simulink model "OMAP"  (R2018b)
settings: Solver=FixedStepDiscrete  StartTime=0.0  StopTime=10.0  FixedStep=0.01  RelTol=1e-3
values from neighbouring files (symbols this model uses):
  Clb_ICADirect_LaneDisp_StateFive = Simulink.Parameter    [omap_ver_442.m]
  Clb_ICADirect_LaneDisp_StateFour = Simulink.Parameter    [omap_ver_442.m]
  Clb_ICADirect_LaneDisp_StateOne = Simulink.Parameter    [omap_ver_442.m]
  Clb_ICADirect_LaneDisp_StateThree = Simulink.Parameter    [omap_ver_442.m]
  Clb_ICADirect_LaneDisp_StateTwo = Simulink.Parameter    [omap_ver_442.m]
  Clb_ICADirect_LaneDisp_StateZero = Simulink.Parameter    [omap_ver_442.m]
  Clb_ICADirect_LaneDispSW = Simulink.Parameter    [omap_ver_442.m]
  Clb_ICADirect_TrnLghtsCom_Switch = Simulink.Parameter    [omap_ver_442.m]
  Clb_ICADirect_TrnLghtsCom_Value = Simulink.Parameter    [omap_ver_442.m]
  Clb_ICADirect_TrnLghtsCrtl_Inhb = Simulink.Parameter    [omap_ver_442.m]
  OMAP_ACCAEB_EMSESC_Decel = Simulink.Parameter    [omap_ver_442.m]
  OMAP_ACCFCW_IC_Decel = Simulink.Parameter    [omap_ver_442.m]
  OMAP_clb_ACC_RVVReqType = Simulink.Parameter    [omap_ver_442.m]
  OMAP_clb_ACC_RVVReqType_Switch = Simulink.Parameter    [omap_ver_442.m]
  OMAP_clb_ACCHeadwayDisplay = Simulink.Parameter    [omap_ver_442.m]
  OMAP_clb_ACCHeadwayDisplay_Switch = Simulink.Parameter    [omap_ver_442.m]
  OMAP_clb_ACCHeadwayIcon = Simulink.Parameter    [omap_ver_442.m]
  OMAP_clb_ACCHeadwayIcon_Switch = Simulink.Parameter    [omap_ver_442.m]
  OMAP_clb_ACCMessagePrompt = Simulink.Parameter    [omap_ver_442.m]
  OMAP_clb_ACCMessagePrompt_Switch = Simulink.Parameter    [omap_ver_442.m]
  OMAP_clb_ACCRequestEPB = Simulink.Parameter    [omap_ver_442.m]
  OMAP_clb_ACCRequestEPB_Switch = Simulink.Parameter    [omap_ver_442.m]
  OMAP_clb_ACCSetSpeed = Simulink.Parameter    [omap_ver_442.m]
  OMAP_clb_ACCSetSpeed_Switch = Simulink.Parameter    [omap_ver_442.m]
  OMAP_clb_ACCSetSpeedDis = Simulink.Parameter    [omap_ver_442.m]
  OMAP_clb_ACCSetSpeedDis_Switch = Simulink.Parameter    [omap_ver_442.m]
  OMAP_clb_ACCState = Simulink.Parameter    [omap_ver_442.m]
  OMAP_clb_ACCState_Switch = Simulink.Parameter    [omap_ver_442.m]
  OMAP_clb_ACCStatusIconDis = Simulink.Parameter    [omap_ver_442.m]
  OMAP_clb_ACCStatusIconDis_Switch = Simulink.Parameter    [omap_ver_442.m]
  OMAP_clb_ACCTorqueReq = Simulink.Parameter    [omap_ver_442.m]
  OMAP_clb_ACCTorqueReq_Switch = Simulink.Parameter    [omap_ver_442.m]
  OMAP_clb_ADAS_State = Simulink.Parameter    [omap_ver_442.m]
  OMAP_clb_ADAS_State_Switch = Simulink.Parameter    [omap_ver_442.m]
  OMAP_clb_AEBAlertReq = Simulink.Parameter    [omap_ver_442.m]
  OMAP_clb_AEBAlertReq_Switch = Simulink.Parameter    [omap_ver_442.m]
  OMAP_clb_AEBBrakingProg = Simulink.Parameter    [omap_ver_442.m]
  OMAP_clb_AEBBrakingProg_Switch = Simulink.Parameter    [omap_ver_442.m]
  OMAP_clb_AEBFaultStatus = Simulink.Parameter    [omap_ver_442.m]
  OMAP_clb_AEBFaultStatus_Switch = Simulink.Parameter    [omap_ver_442.m]
  OMAP_clb_AEBMassageDisp = Simulink.Parameter    [omap_ver_442.m]
  OMAP_clb_AEBMassageDisp_Switch = Simulink.Parameter    [omap_ver_442.m]
  OMAP_clb_AEBState = Simulink.Parameter    [omap_ver_442.m]
  OMAP_clb_AEBState_Switch = Simulink.Parameter    [omap_ver_442.m]
  OMAP_clb_AEBSwitchStatus = Simulink.Parameter    [omap_ver_442.m]
  OMAP_clb_AEBSwitchStatus_Switch = Simulink.Parameter    [omap_ver_442.m]
  OMAP_clb_BrakeRequest = Simulink.Parameter    [omap_ver_442.m]
  OMAP_clb_BrakeRequest_Switch = Simulink.Parameter    [omap_ver_442.m]
  OMAP_clb_DecelerationSet = Simulink.Parameter    [omap_ver_442.m]
  OMAP_clb_DecelerationSet_Switch = Simulink.Parameter    [omap_ver_442.m]
  OMAP_clb_DecelerationType = Simulink.Parameter    [omap_ver_442.m]
  OMAP_clb_DecelerationType_Switch = Simulink.Parameter    [omap_ver_442.m]
  OMAP_clb_DeclControlReq = Simulink.Parameter    [omap_ver_442.m]
  OMAP_clb_DeclControlReq_Switch = Simulink.Parameter    [omap_ver_442.m]
  OMAP_clb_DownorUpGearMinTime = Simulink.Parameter    [omap_ver_442.m]
  OMAP_clb_DownorUpGearMinTime_Switch = Simulink.Parameter    [omap_ver_442.m]
  OMAP_clb_ELKPopupMessage = Simulink.Parameter    [omap_ver_442.m]
  OMAP_clb_ELKPopupMessage_Switch = Simulink.Parameter    [omap_ver_442.m]
  OMAP_clb_ELKSts = Simulink.Parameter    [omap_ver_442.m]
  OMAP_clb_ELKSts_Switch = Simulink.Parameter    [omap_ver_442.m]
  OMAP_clb_ESAFaultSt = Simulink.Parameter    [omap_ver_442.m]
  OMAP_clb_ESAFaultSt_Switch = Simulink.Parameter    [omap_ver_442.m]
  OMAP_clb_ESARequest = Simulink.Parameter    [omap_ver_442.m]
  OMAP_clb_ESARequest_Switch = Simulink.Parameter    [omap_ver_442.m]
  OMAP_clb_ESAState = Simulink.Parameter    [omap_ver_442.m]
  OMAP_clb_ESAState_Switch = Simulink.Parameter    [omap_ver_442.m]
  OMAP_clb_ESATorqueReq = Simulink.Parameter    [omap_ver_442.m]
  OMAP_clb_ESATorqueReq_Switch = Simulink.Parameter    [omap_ver_442.m]
  OMAP_clb_ESCDriveOff = Simulink.Parameter    [omap_ver_442.m]
  OMAP_clb_ESCDriveOff_Switch = Simulink.Parameter    [omap_ver_442.m]
  OMAP_clb_ESCHoldReq = Simulink.Parameter    [omap_ver_442.m]
  OMAP_clb_ESCHoldReq_Switch = Simulink.Parameter    [omap_ver_442.m]
  OMAP_clb_Handsoffwarning = Simulink.Parameter    [omap_ver_442.m]
  OMAP_clb_Handsoffwarning_Switch = Simulink.Parameter    [omap_ver_442.m]
  OMAP_clb_HapticAlarmReq = Simulink.Parameter    [omap_ver_442.m]
  OMAP_clb_HapticAlarmReq_Switch = Simulink.Parameter    [omap_ver_442.m]
  OMAP_clb_HMIPopupMassage = Simulink.Parameter    [omap_ver_442.m]
  OMAP_clb_HMIPopupMassage_Switch = Simulink.Parameter    [omap_ver_442.m]
  OMAP_clb_HWAActionSts = Simulink.Parameter    [omap_ver_442.m]
  OMAP_clb_HWAActionSts_Switch = Simulink.Parameter    [omap_ver_442.m]
  OMAP_clb_HWAMode = Simulink.Parameter    [omap_ver_442.m]
  OMAP_clb_HWAMode_Switch = Simulink.Parameter    [omap_ver_442.m]
  OMAP_clb_HWATurnOnIdctr = Simulink.Parameter    [omap_ver_442.m]
  OMAP_clb_HWATurnOnIdctr_Switch = Simulink.Parameter    [omap_ver_442.m]
  OMAP_clb_ICAMassageDisp = Simulink.Parameter    [omap_ver_442.m]
  OMAP_clb_ICAMassageDisp_Switch = Simulink.Parameter    [omap_ver_442.m]
  OMAP_clb_ICAStatusIcon = Simulink.Parameter    [omap_ver_442.m]
  OMAP_clb_ICAStatusIcon_Switch = Simulink.Parameter    [omap_ver_442.m]
  OMAP_clb_ISLCDriverRemind = Simulink.Parameter    [omap_ver_442.m]
  OMAP_clb_ISLCDriverRemind_Switch = Simulink.Parameter    [omap_ver_442.m]
  OMAP_clb_ISLCState = Simulink.Parameter    [omap_ver_442.m]
  OMAP_clb_ISLCState_Switch = Simulink.Parameter    [omap_ver_442.m]
  OMAP_clb_JAFaultSt = Simulink.Parameter    [omap_ver_442.m]
  OMAP_clb_JAFaultSt_Switch = Simulink.Parameter    [omap_ver_442.m]
  OMAP_clb_LCAPopupMessage = Simulink.Parameter    [omap_ver_442.m]
  OMAP_clb_LCAPopupMessage_Switch = Simulink.Parameter    [omap_ver_442.m]
  OMAP_clb_LCAStatusDisplay = Simulink.Parameter    [omap_ver_442.m]
  OMAP_clb_LCAStatusDisplay_Switch = Simulink.Parameter    [omap_ver_442.m]
  OMAP_clb_LDWStatusDisplay = Simulink.Parameter    [omap_ver_442.m]
  OMAP_clb_LDWStatusDisplay_Switch = Simulink.Parameter    [omap_ver_442.m]
  OMAP_clb_LDWWarningSt = Simulink.Parameter    [omap_ver_442.m]
  OMAP_clb_LDWWarningSt_Switch = Simulink.Parameter    [omap_ver_442.m]
  OMAP_clb_LightControlValid = Simulink.Parameter    [omap_ver_442.m]
  OMAP_clb_LightControlValid_Switch = Simulink.Parameter    [omap_ver_442.m]
  OMAP_clb_LKAActivation = Simulink.Parameter    [omap_ver_442.m]
  OMAP_clb_LKAActivation_Switch = Simulink.Parameter    [omap_ver_442.m]
  OMAP_clb_LKAAngleReq = Simulink.Parameter    [omap_ver_442.m]
  OMAP_clb_LKAAngleReq_Switch = Simulink.Parameter    [omap_ver_442.m]
  OMAP_clb_LKAMode = Simulink.Parameter    [omap_ver_442.m]
  OMAP_clb_LKAMode_Switch = Simulink.Parameter    [omap_ver_442.m]
  OMAP_clb_LKAorELK_CoolTime = Simulink.Parameter    [omap_ver_442.m]
  OMAP_clb_LKAState = Simulink.Parameter    [omap_ver_442.m]
  OMAP_clb_LKAState_Switch = Simulink.Parameter    [omap_ver_442.m]
  OMAP_clb_LKAStatusDisplay = Simulink.Parameter    [omap_ver_442.m]
  OMAP_clb_LKAStatusDisplay_Switch = Simulink.Parameter    [omap_ver_442.m]
  OMAP_clb_LKASwitchState = Simulink.Parameter    [omap_ver_442.m]
  OMAP_clb_LKASwitchState_Switch = Simulink.Parameter    [omap_ver_442.m]
  OMAP_clb_LKATorqFactReq = Simulink.Parameter    [omap_ver_442.m]
  OMAP_clb_LKATorqFactReq_Switch = Simulink.Parameter    [omap_ver_442.m]
  OMAP_clb_PrefillRequest = Simulink.Parameter    [omap_ver_442.m]
  ... (+36 more)
libraries: simulink x184, canmsglib x2
(part 8 of 14)

== system OMAP/Runnable_OMAP_10ms_sys/OMAP_Module/ACCS_Direct/ACCS_Define/Human_Machine_Interface(ACC_HMI) ==
  CIPV_ID_Longitudinal_Distance : Inport
  CIPV_ID : Inport  Port=2
  ACC_State : Inport  Port=3
  ACCActive_Signal : Inport  Port=4
  ACC_ICA_Flag : Inport  Port=5
  HeadWaySet : Inport  Port=6
  VelocitySet : Inport  Port=7
  ACC_go_request : Inport  Port=8
  ACC_DecReq : Inport  Port=9
  Bus Selector : BusSelector  OutputSignals=ACC_Vehicle_Icon_Display,ACC_Set_Speed_Display,ACC_DesiredHeadway_Icon_Basic,RVVACC_Vehiclespeed_request_type
  Gain : Gain  OutDataTypeStr=uint8
  Gain1 : Gain  OutDataTypeStr=uint8
  Subsystem : Subsystem
  Subsystem9 : Subsystem
  Text_PopUp : Subsystem
  ACC_DesiredHeadway_Display : Outport
  ACC_DesiredHeadway_Icon_Basic : Outport  Port=2
  ACC_Desired_Set_Speed : Outport  Port=3
  ACC_Set_Speed_Display : Outport  Port=4
  ACC_Vehicle_Icon_Display : Outport  Port=5
  RVVACC_Vehiclespeed_request_type : Outport  Port=6
  ACC_Pop_Up_Message : Outport  Port=7
  ACC_HMI_TgDisp_Flag : Outport  Port=8
  TARGET_POSITION : Outport  Port=9
  ACC_Pop_Up_Message_TJA : Outport  Port=10
  wires:
  VelocitySet/1 -> Gain/1, Subsystem9/3(VelocitySet)
  HeadWaySet/1 -> Gain1/1
  Subsystem9/1(Out1) -> Bus Selector/1
  Gain/1 -> ACC_Desired_Set_Speed/1  "ACC_Desired_Set_Speed"
  CIPV_ID_Longitudinal_Distance/1 -> Subsystem/1(Distance)
  Subsystem/2(TgDisp_Flag) -> ACC_HMI_TgDisp_Flag/1  "ACC_HMI_TgDisp_Flag"
  Subsystem/1(TARGET_POSITION) -> TARGET_POSITION/1  "TARGET_POSITION"
  CIPV_ID/1 -> Subsystem/2(CIPV_ID)
  Gain1/1 -> ACC_DesiredHeadway_Display/1  "ACC_DesiredHeadway_Display"
  Text_PopUp/1(For4F7) -> ACC_Pop_Up_Message/1  "ACC_Pop_Up_Message"
  Bus Selector/1 -> ACC_Vehicle_Icon_Display/1  "<ACC_Vehicle_Icon_Display>"
  Bus Selector/3 -> ACC_DesiredHeadway_Icon_Basic/1  "<ACC_DesiredHeadway_Icon_Basic>"
  Bus Selector/4 -> RVVACC_Vehiclespeed_request_type/1  "<RVVACC_Vehiclespeed_request_type>"
  Bus Selector/2 -> ACC_Set_Speed_Display/1  "<ACC_Set_Speed_Display>"
  ACCActive_Signal/1 -> Text_PopUp/3(ACCActive_Signal)
  Text_PopUp/2(ForTJA) -> ACC_Pop_Up_Message_TJA/1  "ACC_Pop_Up_Message_TJA"
  ACC_go_request/1 -> Text_PopUp/4(go_request)
  ACC_State/1 -> Subsystem9/1(ACC_State), Text_PopUp/1(ACC_State), Subsystem/3(ACC_State)
  ACC_ICA_Flag/1 -> Subsystem9/2(ACCICA_Flag), Text_PopUp/2(ACCICA_Flag)
  ACC_DecReq/1 -> Text_PopUp/5(ACC_DecReq)

== system OMAP/Runnable_OMAP_10ms_sys/OMAP_Module/ICA_Direct_G59/ICA_Define/ICA_EPS ==
  EPSPCEM_stICAState : Inport
  angle : Inport  Port=2
  torque_Req : Inport  Port=3
  torque : Inport  Port=4
  EPSPCEM_stEPSCtlState : Inport  Port=5
  Data Type Conversion : DataTypeConversion  OutDataTypeStr=uint16
  Data Type Conversion1 : DataTypeConversion  OutDataTypeStr=single
  Data Type Conversion2 : DataTypeConversion  OutDataTypeStr=uint16
  Data Type Conversion3 : DataTypeConversion  OutDataTypeStr=single
  Data Type Conversion4 : DataTypeConversion  OutDataTypeStr=single
  EPS_Ctr_Disable : Subsystem  TreatAsAtomicUnit=on
  EPS_Ctr_Enable : Subsystem  TreatAsAtomicUnit=on
  If1 : If  IfExpression=u1==3
  Merge{1..5} (5 alike) : Merge
  stEPS_State_Ctl_CMD : Outport
  LKA_TRQ_FACT_REQ : Outport  Port=2
  LKA_OR_LPA_REQ : Outport  Port=3
  ICA_STATE : Outport  Port=4
  ICABve_g_SteerAngleCmd_convert : Outport  Port=5
  ICABve_d_LKATorqueReq_convert : Outport  Port=6
  ICABve_g_LKATorqueReq_Value_convert : Outport  Port=7
  wires:
  Merge1/1 -> Data Type Conversion/1
  EPSPCEM_stEPSCtlState/1 -> EPS_Ctr_Disable/1(stEPSCtlState), EPS_Ctr_Enable/1(stEPSCtlState)
  EPS_Ctr_Enable/1(stEPSCtlCMD) -> Merge1/1
  If1/2 -> EPS_Ctr_Disable/Action
  EPS_Ctr_Enable/2(LKA_TRQ_FACT_REQ) -> Merge2/1
  EPS_Ctr_Disable/2(LKA_TRQ_FACT_REQ) -> Merge2/2
  Merge2/1 -> Data Type Conversion1/1
  EPSPCEM_stICAState/1 -> ICA_STATE/1, If1/1
  Data Type Conversion1/1 -> LKA_TRQ_FACT_REQ/1  "LKA_TRQ_FACT_REQ"
  EPS_Ctr_Disable/1(stEPSCtlCMD) -> Merge1/2
  If1/1 -> EPS_Ctr_Enable/Action
  Data Type Conversion/1 -> stEPS_State_Ctl_CMD/1
  EPS_Ctr_Enable/3(LKA_OR_LPA_REQ) -> Merge3/1
  Data Type Conversion2/1 -> LKA_OR_LPA_REQ/1
  Merge3/1 -> Data Type Conversion2/1
  EPS_Ctr_Disable/3(LKA_OR_LPA_REQ) -> Merge3/2
  Data Type Conversion3/1 -> ICABve_g_SteerAngleCmd_convert/1
  Merge5/1 -> Data Type Conversion4/1
  Merge4/1 -> Data Type Conversion3/1
  Data Type Conversion4/1 -> ICABve_g_LKATorqueReq_Value_convert/1
  EPS_Ctr_Disable/5(torque1) -> Merge5/2
  EPS_Ctr_Disable/4(angle1) -> Merge4/2
  angle/1 -> EPS_Ctr_Enable/2(angle)
  torque/1 -> EPS_Ctr_Enable/3(torque)
  EPS_Ctr_Enable/4(angle1) -> Merge4/1
  EPS_Ctr_Enable/5(torque1) -> Merge5/1
  torque_Req/1 -> ICABve_d_LKATorqueReq_convert/1

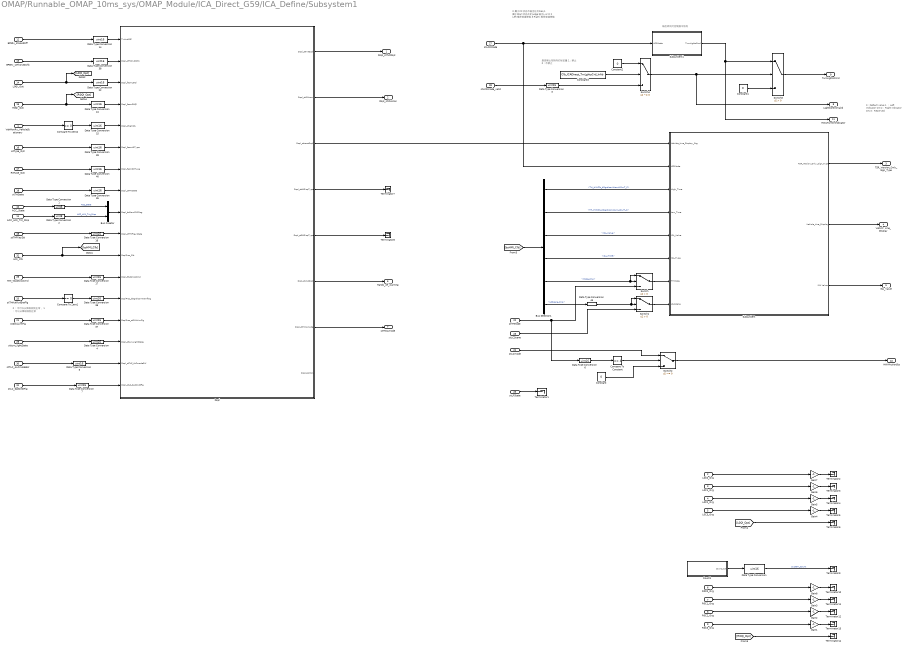
== system OMAP/Runnable_OMAP_10ms_sys/OMAP_Module/ICA_Direct_G59/ICA_Define/Subsystem1 ==
  note: 是否禁止控转向灯标定量
      | 1：禁止
      | 0：不禁止
  note: 0：Default value
      | 1：Left indicator ON
      | 2：Right indicator ON
      | 3：Reserved
  note: 输出转向灯控制指令信号
  note: 0 ：不可以从降级回到正常，
      | 1 ：可以从降级回到正常
  note: 0 属于CD状态不输出任何Req
      | 1 属于Start状态开始Judge输出L or R
      | 2 Left推荐变道使能
      | 3 Right 推荐变道使能
  VehMovRx_VehicleStationary : Inport
  L0C0_Org : Inport  Port=2
  L0C1_Org : Inport  Port=3
  L0C2_Org : Inport  Port=4
  L0C3_Org : Inport  Port=5
  R0C0_Org : Inport  Port=6
  R0C1_Org : Inport  Port=7
  R0C2_Org : Inport  Port=8
  R0C3_Org : Inport  Port=9
  ACC_State : Inport  Port=10
  ACC_HMI_Txt_Disp : Inport  Port=11
  EPSRx_stHandOff : Inport  Port=12
  EPSRx_stTkOvStChk : Inport  Port=13
  L0QI_Opt : Inport  Port=14
  R0QI_Opt : Inport  Port=15
  L0Type_Opt : Inport  Port=16
  R0Type_Opt : Inport  Port=17
  stTHState : Inport  Port=18
  stTHFKeyStt : Inport  Port=19
  stTHAutRydEnaFlg : Inport  Port=20
  stSWALimFlg : Inport  Port=21
  stTHMode : Inport  Port=22
  stLCScene : Inport  Port=23
  stLCmode : Inport  Port=24
  stLFState : Inport  Port=25
  HMI_tfAddVocCmd : Inport  Port=26
  stLCRMode : Inport  Port=27
  stLCRmode_valid : Inport  Port=28
  stturn_lightState : Inport  Port=29
  stTLC_ALCmodeSW : Inport  Port=30
  stLC_SpdCndtFlg : Inport  Port=31
  HMI_Clb : Inport  Port=32
  Bus Creator : BusCreator  Inputs=2
  Bus Selector1 : BusSelector  OutputSignals=TH_HMIClb_tiDgrdIconWarnHiDurT_C,TH_HMIClb_tiDgrdIconWarnLoDurT_C,ISA_Value,ISA_TYPE,Mode_tmp,LCScene_tmp
  Compare To Constant : simulink/Logic and Bit Operations/Compare To Constant  relop===  const=4  OutDataTypeStr=boolean
  Compare To Zero1 : simulink/Logic and Bit Operations/Compare To Zero  relop===  OutDataTypeStr=boolean
  Compare To Zero2 : simulink/Logic and Bit Operations/Compare To Zero  relop===  OutDataTypeStr=boolean
  Constant : Constant  Value=0  OutDataTypeStr=uint16
  Constant1 : Constant  Value=0  OutDataTypeStr=uint16
  Constant2 : Constant  Value=0  OutDataTypeStr=uint16
  Constant3 : Constant  Value=Clb_ICADirect_TrnLghtsCrtl_Inhb  OutDataTypeStr=uint16
  Count1 : MATLAB Function  TreatAsAtomicUnit=on
  Data Type Conversion{,3..7,14..17,22,24,35..40,45} (19 alike) : DataTypeConversion  OutDataTypeStr=uint16
  Data Type Conversion1 : DataTypeConversion  OutDataTypeStr=uint8
  Data Type Conversion2 : DataTypeConversion  OutDataTypeStr=uint8
  Dspl : Subsystem
  Gain{1..8} (8 alike) : Gain  Gain=-1  OutDataTypeStr=single
  Subsystem : Subsystem
  Subsystem1 : Subsystem
  Switch : Switch  Criteria=u2 > Threshold  OutDataTypeStr=uint16
  Switch1 : Switch  Criteria=u2 > Threshold  OutDataTypeStr=uint16
  Switch2 : Switch  Criteria=u2 ~= 0  OutDataTypeStr=uint16
  Switch3 : Switch  Criteria=u2 > Threshold  OutDataTypeStr=uint16
  Switch4 : Switch  Criteria=u2 ~= 0
  Terminator{1..14} (14 alike) : Terminator
  Dspl_stTxtDspl : Outport
  Dspl_stICAIcon : Outport  Port=2
  TSR_Version_Only_Sign_Type : Outport  Port=3
  Vehiclr_Line_Display : Outport  Port=4
  ISA_Value : Outport  Port=5
  Hands_off_warning : Outport  Port=6
  stHWAmode : Outport  Port=7
  LightControlValid : Outport  Port=8
  TurnLightsCmd : Outport  Port=9
  HWAActionSts : Outport  Port=10
  HWATurnOnIndicator : Outport  Port=11
  wires:
  R0C3_Org/1 -> Gain1/1
  L0C0_Org/1 -> Gain7/1
  stTHFKeyStt/1 -> Data Type Conversion16/1
  [L0QI_Opt] -> Terminator6/1
  Dspl/6(Dspl_stVocDspl) -> Hands_off_warning/1
  stLCScene/1 -> Switch1/3
  stTHMode/1 -> Data Type Conversion6/1, Switch/3
  L0QI_Opt/1 -> [L0QI_Opt], Data Type Conversion22/1
  stTHAutRydEnaFlg/1 -> Compare To Zero1/1
  stTHState/1 -> Data Type Conversion35/1
  stSWALimFlg/1 -> Data Type Conversion37/1
  [R0QI_Opt] -> Terminator14/1
  R0C0_Org/1 -> Gain8/1
  L0C2_Org/1 -> Gain5/1
  R0Type_Opt/1 -> Data Type Conversion40/1
  VehMovRx_VehicleStationary/1 -> Compare To Zero2/1
  Data Type Conversion24/1 -> Dspl/4(Dspl_facmR0Ql)
  R0QI_Opt/1 -> [R0QI_Opt], Data Type Conversion24/1
  R0C1_Org/1 -> Gain3/1
  Compare To Zero1/1 -> Data Type Conversion36/1
  Data Type Conversion39/1 -> Dspl/6(Dspl_facmL0Type)
  Data Type Conversion37/1 -> Dspl/14(DsplPrcs_stSWALimFlg)
  L0C3_Org/1 -> Gain4/1
  Data Type Conversion17/1 -> Dspl/12(Dspl_tfAddVocCmd)
  Bus Selector1/6 -> Data Type Conversion45/1  "<LCScene_tmp>"
  Data Type Conversion16/1 -> Dspl/10(Dspl_stTHFKeyState)
  EPSRx_stTkOvStChk/1 -> Data Type Conversion38/1
  [bsHMI_Clb] -> Bus Selector1/1
  Data Type Conversion45/1 -> Switch1/1, Switch1/2
  Data Type Conversion36/1 -> Dspl/13(DsplPrcs_dDgrdIconWarnflag)
  HMI_Clb/1 -> [bsHMI_Clb], Dspl/11(DsplPrcs_CIb)
  Data Type Conversion40/1 -> Dspl/7(Dspl_facmR0Type)
  Bus Selector1/2 -> Subsystem/4(Low_Time)  "<TH_HMIClb_tiDgrdIconWarnLoDurT_C>"
  Count1/1(count_out) -> Data Type Conversion/1
  EPSRx_stHandOff/1 -> Data Type Conversion14/1
  Dspl/3(Dspl_stLaneDspl) -> Subsystem/1(Vehicle_Line_Display_Org)
  Switch/1 -> Subsystem/7(THMode)
  Data Type Conversion22/1 -> Dspl/3(Dspl_facmL0Ql)
  Data Type Conversion15/1 -> Dspl/5(Dspl_stVehSty)
  Dspl/5(Dspl_stR0DispType) -> Terminator8/1
  Data Type Conversion35/1 -> Dspl/8(Dspl_stTHState)
  Data Type Conversion14/1 -> Dspl/1(TxHndOff)
  Dspl/4(Dspl_stL0DispType) -> Terminator7/1
  L0C1_Org/1 -> Gain6/1
  L0Type_Opt/1 -> Data Type Conversion39/1
  Bus Selector1/1 -> Subsystem/3(High_Time)  "<TH_HMIClb_tiDgrdIconWarnHiDurT_C>"
  Gain2/1 -> Terminator12/1
  Gain3/1 -> Terminator11/1
  Gain7/1 -> Terminator2/1
  R0C2_Org/1 -> Gain2/1
  Gain6/1 -> Terminator3/1
  Gain5/1 -> Terminator4/1
  Gain8/1 -> Terminator10/1
  Switch1/1 -> Subsystem/8(LC_Scene)
  Gain1/1 -> Terminator13/1
  HMI_tfAddVocCmd/1 -> Data Type Conversion17/1
  Subsystem/1(TSR_Version_Only_Sign_Type) -> TSR_Version_Only_Sign_Type/1
  Bus Selector1/3 -> Subsystem/5(ISA_Value)  "<ISA_Value>"
  Subsystem/3(ISA Value) -> ISA_Value/1
  Bus Selector1/4 -> Subsystem/6(ISA_Type)  "<ISA_TYPE>"
  Subsystem/2(Vehicle_Line_Display) -> Vehiclr_Line_Display/1
  Data Type Conversion38/1 -> Dspl/2(Dspl_stTkOvStChk)
  Data Type Conversion/1 -> Terminator9/1  "System_Count"
  Gain4/1 -> Terminator5/1
  Bus Selector1/5 -> Switch/1, Switch/2  "<Mode_tmp>"
  Bus Creator/1 -> Dspl/9(Dspl_bsFromFMCMsg)
  Data Type Conversion2/1 -> Bus Creator/2  "ACC_HMI_Txt_Disp"
  Data Type Conversion1/1 -> Bus Creator/1  "ACC_State"
  ACC_HMI_Txt_Disp/1 -> Data Type Conversion2/1
  ACC_State/1 -> Data Type Conversion1/1
  Dspl/1(Dspl_stTxtDspl) -> Dspl_stTxtDspl/1
  Dspl/2(Dspl_stICAIcon) -> Dspl_stICAIcon/1
  Subsystem1/1(TurnLightsCmd) -> HWATurnOnIndicator/1, Switch3/1
  Compare To Zero2/1 -> Data Type Conversion15/1
  stLCmode/1 -> Switch2/1
  stLFState/1 -> Terminator1/1
  stLCRmode_valid/1 -> Data Type Conversion3/1
  stturn_lightState/1 -> Data Type Conversion4/1
  stTLC_ALCmodeSW/1 -> Data Type Conversion5/1
  Data Type Conversion4/1 -> Dspl/15(Dspl_stturn_lightState)
  Data Type Conversion5/1 -> Dspl/16(Dspl_stTLC_ALCmodeSW)
  Data Type Conversion6/1 -> Compare To Constant/1
  Compare To Constant/1 -> Switch2/2
  Constant/1 -> Switch2/3
  Switch2/1 -> HWAActionSts/1
  stLC_SpdCndtFlg/1 -> Data Type Conversion7/1
  Data Type Conversion7/1 -> Dspl/17(Dspl_stLC_SpdCndtFlg)
  Dspl/7(Dspl_stHWAmode) -> stHWAmode/1
  Switch3/1 -> TurnLightsCmd/1
  Constant1/1 -> Switch3/3
  stLCRMode/1 -> Subsystem1/1(LCRMode), Subsystem/2(LCRMode)
  Data Type Conversion3/1 -> Switch4/3
  Switch4/1 -> LightControlValid/1, Switch3/2
  Constant2/1 -> Switch4/1
  Constant3/1 -> Switch4/2

== system OMAP/Runnable_OMAP_10ms_sys/OMAP_Module/ICA_Direct_G59/ICA_Define/TH_HMIClb ==
  note: Level: 3
      | Num: THC.06
      | Rev: 00.00.01
      | Ud: 19-03-28
  Bus Creator1 : BusCreator  Inputs=15
  Constant : Constant  Value=0.01  OutDataTypeStr=single
  Data Type Conversion{,1..7} (8 alike) : DataTypeConversion  OutDataTypeStr=single
  Data Type Conversion{10..13} (4 alike) : DataTypeConversion  OutDataTypeStr=uint16
  ISA_TYPE : Subsystem
      mask Display:
      | port_label('input', 1, 'In');
      | port_label('output', 1, 'Out');
      | color('blue');
      | text(0.5,0.5,'0.789','horizontalAlignment','center');
  ISA_Value : Subsystem
      mask Display:
      | port_label('input', 1, 'In');
      | port_label('output', 1, 'Out');
      | color('blue');
      | text(0.5,0.5,'0.789','horizontalAlignment','center');
  LCScene_tmp : Subsystem
      mask Display:
      | port_label('input', 1, 'In');
      | port_label('output', 1, 'Out');
      | color('blue');
      | text(0.5,0.5,'0.789','horizontalAlignment','center');
  Mode_tmp : Subsystem
      mask Display:
      | port_label('input', 1, 'In');
      | port_label('output', 1, 'Out');
      | color('blue');
      | text(0.5,0.5,'0.789','horizontalAlignment','center');
  TH_HMIClb_tiDgrdIconWarnHiDurT_C : Subsystem
      mask Display:
      | port_label('input', 1, 'In');
      | port_label('output', 1, 'Out');
      | color('blue');
      | text(0.5,0.5,'0.789','horizontalAlignment','center');
  TH_HMIClb_tiDgrdIconWarnLoDurT_C : Subsystem
      mask Display:
      | port_label('input', 1, 'In');
      | port_label('output', 1, 'Out');
      | color('blue');
      | text(0.5,0.5,'0.789','horizontalAlignment','center');
  TH_HMIClb_tiDgrdVocWarnDurT_C : Subsystem
      mask Display:
      | port_label('input', 1, 'In');
      | port_label('output', 1, 'Out');
      | color('blue');
      | text(0.5,0.5,'0.789','horizontalAlignment','center');
  "TH_HMIClb_tiHndOffTxtWarnT_C " : Subsystem
      mask Display:
      | port_label('input', 1, 'In');
      | port_label('output', 1, 'Out');
      | color('blue');
      | text(0.5,0.5,'0.789','horizontalAlignment','center');
  TH_HMIClb_tiHndOffVocWarnT_C : Subsystem
      mask Display:
      | port_label('input', 1, 'In');
      | port_label('output', 1, 'Out');
      | color('blue');
      | text(0.5,0.5,'0.789','horizontalAlignment','center');
  TH_HMIClb_tiSWALimFlgDetT_C : Subsystem
      mask Display:
      | port_label('input', 1, 'In');
      | port_label('output', 1, 'Out');
      | color('blue');
      | text(0.5,0.5,'0.789','horizontalAlignment','center');
  TH_HMIClb_tiTxtLimT_C : Subsystem
      mask Display:
      | port_label('input', 1, 'In');
      | port_label('output', 1, 'Out');
      | color('blue');
      | text(0.5,0.5,'0.789','horizontalAlignment','center');
  Out : Outport
  wires:
  Bus Creator1/1 -> Out/1
  "TH_HMIClb_tiHndOffTxtWarnT_C "/1(Out1) -> Bus Creator1/1  "TH_HMIClb_tiHndOffTxtWarnT_C"
  Data Type Conversion3/1 -> "TH_HMIClb_tiHndOffTxtWarnT_C "/1(In2)
  TH_HMIClb_tiHndOffVocWarnT_C/1(Out1) -> Bus Creator1/2  "TH_HMIClb_tiHndOffVocWarnT_C"
  Data Type Conversion1/1 -> TH_HMIClb_tiHndOffVocWarnT_C/1(In2)
  TH_HMIClb_tiDgrdVocWarnDurT_C/1(Out1) -> Bus Creator1/3  "TH_HMIClb_tiDgrdVocWarnDurT_C"
  Data Type Conversion2/1 -> TH_HMIClb_tiDgrdVocWarnDurT_C/1(In2)
  TH_HMIClb_tiTxtLimT_C/1(Out1) -> Bus Creator1/4  "TH_HMIClb_tiTxtLimT_C"
  Data Type Conversion4/1 -> TH_HMIClb_tiTxtLimT_C/1(In2)
  Data Type Conversion/1 -> Bus Creator1/5  "TH_HMIClb_tiCalcPer_C"
  TH_HMIClb_tiDgrdIconWarnHiDurT_C/1(Out1) -> Bus Creator1/6  "TH_HMIClb_tiDgrdIconWarnHiDurT_C"
  Data Type Conversion5/1 -> TH_HMIClb_tiDgrdIconWarnHiDurT_C/1(In2)
  TH_HMIClb_tiDgrdIconWarnLoDurT_C/1(Out1) -> Bus Creator1/7  "TH_HMIClb_tiDgrdIconWarnLoDurT_C"
  Data Type Conversion6/1 -> TH_HMIClb_tiDgrdIconWarnLoDurT_C/1(In2)
  TH_HMIClb_tiSWALimFlgDetT_C/1(Out1) -> Bus Creator1/8  "TH_HMIClb_tiSWALimFlgDetT_C"
  Data Type Conversion7/1 -> TH_HMIClb_tiSWALimFlgDetT_C/1(In2)
  LCScene_tmp/1(Out1) -> Bus Creator1/11  "LCScene_tmp"
  Data Type Conversion10/1 -> LCScene_tmp/1(In2)  "LCScene_tmp"
  Data Type Conversion12/1 -> ISA_TYPE/1(In2)  "ISA_TYPE"
  ISA_TYPE/1(Out1) -> Bus Creator1/13  "ISA_TYPE"
  ISA_Value/1(Out1) -> Bus Creator1/14  "ISA_Value"
  Data Type Conversion13/1 -> ISA_Value/1(In2)  "ISA_Value"
  Mode_tmp/1(Out1) -> Bus Creator1/15  "Mode_tmp"
  Data Type Conversion11/1 -> Mode_tmp/1(In2)
  Constant/1 -> Data Type Conversion/1

== system OMAP/Runnable_OMAP_10ms_sys/OMAP_Module/Subsystem/EMS_Arbitration/ACC//ICA_arb_AEB//JA ==
  note: 仲裁#3——ACC/ICA与AEB/JAEB
      | 1. 当ACC/ICA在控车且造成的实车减速度已达到（标定值暂定-2.3），若AEB只触发第一档刹车（-2），则仍以ACC/ICA优先。实时监测运算，以当前周期的实车减速度数值为准。
      | 2. 若AEB进一步触发了第二档刹车（-2以上），或者触发了JAEB刹车（总共就一档，-2以上），则AEB/JAEB根据自身的运算正常触发，无条件优先于ACC/ICA
  Input_ACCS : Inport
  Input_AEBS : Inport  Port=2
  Input_JABS : Inport  Port=3
  Input_IMAP : Inport  Port=4
  AEB_arb_JA : Subsystem
  Bus Creator2 : BusCreator  Inputs=5
  Bus Selector : BusSelector  OutputSignals=IMAPve_g_ESC_LonAcc_convert
  Bus Selector2 : BusSelector  OutputSignals=actuator.Function_Acc_status,actuator.PotACCTqReq,actuator.ACCTqReq,actuator.Powertrain_torquewheel_request,actuator.TminUpGear,actuator.StAcvTqWhlPTPotReq
  Compare To Constant : simulink/Logic and Bit Operations/Compare To Constant  relop=>=  const=OMAP_ACCAEB_EMSESC_Decel  OutDataTypeStr=boolean
  Compare To Constant3 : simulink/Logic and Bit Operations/Compare To Constant  relop===  const=4  OutDataTypeStr=boolean
  Compare To Constant4 : simulink/Logic and Bit Operations/Compare To Constant  relop===  const=6  OutDataTypeStr=boolean
  Compare To Constant5 : simulink/Logic and Bit Operations/Compare To Constant  relop=~=  const=4  OutDataTypeStr=boolean
  Compare To Constant6 : simulink/Logic and Bit Operations/Compare To Constant  relop=~=  const=6  OutDataTypeStr=boolean
  Data Type Conversion1 : DataTypeConversion  OutDataTypeStr=single
  Data Type Conversion2 : DataTypeConversion  OutDataTypeStr=uint8
  Data Type Conversion3 : DataTypeConversion  OutDataTypeStr=single
  Data Type Conversion4 : DataTypeConversion  OutDataTypeStr=uint8
  Data Type Conversion61 : DataTypeConversion  OutDataTypeStr=single
  Logical Operator1 : Logic  AllPortsSameDT=off  OutDataTypeStr=boolean
  Logical Operator2 : Logic  Operator=OR  AllPortsSameDT=off  OutDataTypeStr=boolean
  Logical Operator3 : Logic  AllPortsSameDT=off  OutDataTypeStr=boolean
  Logical Operator4 : Logic  Operator=OR  AllPortsSameDT=off  OutDataTypeStr=boolean
  Logical Operator5 : Logic  AllPortsSameDT=off  OutDataTypeStr=boolean
  Switch : Switch  Criteria=u2 ~= 0
  Switch1 : Switch  Criteria=u2 ~= 0
  Out1 : Outport
  Function_Acc_status : Outport  Port=2
  wires:
  Data Type Conversion61/1 -> Bus Creator2/1  "OMAPve_g_PotACCTqReq_1"
  Bus Creator2/1 -> Switch1/3
  Switch1/1 -> Switch/3
  Data Type Conversion2/1 -> Bus Creator2/3  "OMAPve_y_Powertrain_torquewheel_request_1"
  Bus Selector2/2 -> Data Type Conversion61/1  "<PotACCTqReq>"
  Bus Selector/1 -> Compare To Constant/1  "<IMAPve_g_ESC_LonAcc_convert>"
  Input_ACCS/1 -> Bus Selector2/1
  Bus Selector2/4 -> Data Type Conversion2/1  "<Powertrain_torquewheel_request>"
  Data Type Conversion1/1 -> Bus Creator2/2  "OMAPve_g_ACCTqReq_1"
  Input_AEBS/1 -> AEB_arb_JA/1(Input_AEBS)
  AEB_arb_JA/2(Out2) -> Switch/2
  Input_JABS/1 -> AEB_arb_JA/2(Input_JABS)
  AEB_arb_JA/1(Out1) -> Switch1/1, Switch/1
  AEB_arb_JA/3(Out3) -> Logical Operator1/1
  Bus Selector2/5 -> Data Type Conversion3/1  "<TminUpGear>"
  Bus Selector2/3 -> Data Type Conversion1/1  "<ACCTqReq>"
  Data Type Conversion4/1 -> Bus Creator2/5  "OMAPve_y_stAcvTqWhlPTPotReq_1"
  Bus Selector2/6 -> Data Type Conversion4/1  "<StAcvTqWhlPTPotReq>"
  Data Type Conversion3/1 -> Bus Creator2/4  "OMAPve_g_TminUp_or_downGear_1"
  Bus Selector2/1 -> Compare To Constant5/1, Compare To Constant6/1, Compare To Constant3/1, Compare To Constant4/1, Function_Acc_status/1  "<Function_Acc_status>"
  Switch/1 -> Out1/1
  Input_IMAP/1 -> Bus Selector/1
  Logical Operator1/1 -> Switch1/2
  Compare To Constant/1 -> Logical Operator3/2
  Logical Operator2/1 -> Logical Operator1/2
  Logical Operator3/1 -> Logical Operator2/2
  Compare To Constant6/1 -> Logical Operator5/2
  Logical Operator5/1 -> Logical Operator2/1
  Logical Operator4/1 -> Logical Operator3/1
  Compare To Constant3/1 -> Logical Operator4/1
  Compare To Constant5/1 -> Logical Operator5/1
  Compare To Constant4/1 -> Logical Operator4/2

== system OMAP/Runnable_OMAP_10ms_sys/OMAP_Module/Subsystem/EMS_Arbitration/FAPA_arb_ADAS ==
  note: 仲裁#21——FAPA与ADAS
      | 1. 关于EMS、ESC、EPS执行器控制：FAPA在控制车辆的工作阶段，无条件优先于ADAS各个功能；在其他情况，则直连ADAS内部原本的仲裁结果
      | 2. 关于仪表显示：维持原本的仲裁策略
      | 3. 选用的表征信号，经IMAP转译后为IMAPve_d_APA_AutoPark_WorkSt
  Input_ACCICAAEBJA : Inport
  Input_ACCstatus : Inport  Port=2
  Input_FAPA : Inport  Port=3
  Bus Creator : BusCreator  Inputs=7
  Bus Creator1 : BusCreator  Inputs=7
  Bus Selector : BusSelector  OutputSignals=IMAPve_d_APA_AutoPark_WorkSt
  Bus Selector5 : BusSelector  OutputSignals=OMAPve_g_PotACCTqReq_1,OMAPve_g_ACCTqReq_1,OMAPve_y_Powertrain_torquewheel_request_1,OMAPve_g_TminUp_or_downGear_1,OMAPve_y_stAcvTqWhlPTPotReq_1
  Data Type Conversion : DataTypeConversion  OutDataTypeStr=uint8
  OMAPve_g_ACCTqReqNum : Constant  Value=-4000  OutDataTypeStr=single
  OMAPve_g_PotACCTqReqNum : Constant  Value=-4000  OutDataTypeStr=single
  OMAPve_g_TminUp_or_downGearNum : Constant  Value=6.2  OutDataTypeStr=single
  OMAPve_y_ACC_Engine_Start_RequestNum : Constant  Value=0  OutDataTypeStr=uint8
  OMAPve_y_ACC_Engine_Start_RequestNum1 : Constant  Value=0  OutDataTypeStr=uint8
  OMAPve_y_Function_Acc_statusNum : Constant  Value=3  OutDataTypeStr=uint8
  OMAPve_y_Powertrain_torquewheel_requestNum : Constant  Value=0  OutDataTypeStr=uint8
  OMAPve_y_stAcvTqWhlPTPotReqNum : Constant  Value=0  OutDataTypeStr=uint8
  Switch : Switch  Criteria=u2 ~= 0
  Arbitration_EMS : Outport
  wires:
  Bus Selector5/3 -> Bus Creator1/4  "<OMAPve_y_Powertrain_torquewheel_request_1>"
  Bus Selector5/2 -> Bus Creator1/3  "<OMAPve_g_ACCTqReq_1>"
  Bus Selector5/1 -> Bus Creator1/2  "<OMAPve_g_PotACCTqReq_1>"
  Data Type Conversion/1 -> Bus Creator1/7  "OMAPve_y_Function_Acc_status_1"
  Input_FAPA/1 -> Bus Selector/1
  Bus Selector5/5 -> Bus Creator1/6  "<OMAPve_y_stAcvTqWhlPTPotReq_1>"
  Bus Selector5/4 -> Bus Creator1/5  "<OMAPve_g_TminUp_or_downGear_1>"
  OMAPve_y_ACC_Engine_Start_RequestNum1/1 -> Bus Creator1/1  "OMAPve_y_ACC_Engine_Start_Request_1"
  Input_ACCstatus/1 -> Data Type Conversion/1
  Switch/1 -> Arbitration_EMS/1  "Arbitration_EMS"
  Input_ACCICAAEBJA/1 -> Bus Selector5/1
  OMAPve_y_ACC_Engine_Start_RequestNum/1 -> Bus Creator/1  "OMAPve_y_ACC_Engine_Start_Request_1"
  OMAPve_g_TminUp_or_downGearNum/1 -> Bus Creator/5  "OMAPve_g_TminUp_or_downGear_1"
  OMAPve_y_stAcvTqWhlPTPotReqNum/1 -> Bus Creator/6  "OMAPve_y_stAcvTqWhlPTPotReq_1"
  OMAPve_g_ACCTqReqNum/1 -> Bus Creator/3  "OMAPve_g_ACCTqReq_1"
  OMAPve_y_Powertrain_torquewheel_requestNum/1 -> Bus Creator/4  "OMAPve_y_Powertrain_torquewheel_request_1"
  OMAPve_y_Function_Acc_statusNum/1 -> Bus Creator/7  "OMAPve_y_Function_Acc_status_1"
  OMAPve_g_PotACCTqReqNum/1 -> Bus Creator/2  "OMAPve_g_PotACCTqReq_1"
  Bus Selector/1 -> Switch/2  "<IMAPve_d_APA_AutoPark_WorkSt>"
  Bus Creator/1 -> Switch/1  "LKA_EMS"
  Bus Creator1/1 -> Switch/3  "Arbitration_EMS"

== system OMAP/Runnable_OMAP_10ms_sys/OMAP_Module/Subsystem/EPS_Default_Arbitration/AEB//JA_arb_ELK ==
  note: 仲裁#8——AEB/FCW/JAEB/JACW与ELK
      | 1.AEB/FCW/JAEB/JACW无条件优先于ELK
  In1 : Inport
  In2 : Inport  Port=2
  In3 : Inport  Port=3
  Bus Creator : BusCreator  Inputs=4
  Bus Selector1 : BusSelector  OutputSignals=ELKSve_y_EPS_State_Control_convert,ELKSve_g_EPS_Factor_Control_convert,ELKSve_g_ELK_SWA_Control_convert,ELKSve_y_EPS_ELK_Control_convert
  Bus Selector2 : BusSelector  OutputSignals=AEBSve_d_AEBAlertReq_convert
  Bus Selector4 : BusSelector  OutputSignals=JABSve_d_DbAlertReq_convert
  Compare To Constant : simulink/Logic and Bit Operations/Compare To Constant  relop=~=  const=0  OutDataTypeStr=boolean
  Compare To Constant4 : simulink/Logic and Bit Operations/Compare To Constant  relop=~=  const=0  OutDataTypeStr=boolean
  Index Vector1 : MultiPortSwitch  DataPortOrder=Zero-based contiguous  Inputs=2  zeroidx=on  OutDataTypeStr=uint8
  Index Vector2 : MultiPortSwitch  DataPortOrder=Zero-based contiguous  Inputs=2  zeroidx=on  OutDataTypeStr=single
  Index Vector3 : MultiPortSwitch  DataPortOrder=Zero-based contiguous  Inputs=2  zeroidx=on  OutDataTypeStr=single
  Index Vector4 : MultiPortSwitch  DataPortOrder=Zero-based contiguous  Inputs=2  zeroidx=on  OutDataTypeStr=uint8
  Logical Operator1 : Logic  Operator=OR  AllPortsSameDT=off  OutDataTypeStr=boolean
  OMAPve_g_Coefficient_toregulate_EPSNum : Constant  Value=0  OutDataTypeStr=single
  OMAPve_g_Column_angle_setpoint3F2Num : Constant  Value=0  OutDataTypeStr=single
  OMAPve_y_General_state_of_LKA_function3F2Num : Constant  Value=0  OutDataTypeStr=uint8
  OMAPve_y_Permit_to_know_if_LKA_or_LPA3F2Num : Constant  Value=0  OutDataTypeStr=uint8
  Out1 : Outport
  wires:
  Bus Selector1/2 -> Index Vector2/2  "<ELKSve_g_EPS_Factor_Control_convert>"
  Bus Selector1/1 -> Index Vector1/2  "<ELKSve_y_EPS_State_Control_convert>"
  Bus Selector1/4 -> Index Vector4/2  "<ELKSve_y_EPS_ELK_Control_convert>"
  Index Vector4/1 -> Bus Creator/4  "OMAPve_y_Permit_to_know_if_LKA_or_LPA3F2_2"
  OMAPve_g_Coefficient_toregulate_EPSNum/1 -> Index Vector2/3  "OMAPve_g_Coefficient_toregulate_EPS_2"
  Logical Operator1/1 -> Index Vector1/1, Index Vector2/1, Index Vector3/1, Index Vector4/1
  OMAPve_y_Permit_to_know_if_LKA_or_LPA3F2Num/1 -> Index Vector4/3  "OMAPve_y_Permit_to_know_if_LKA_or_LPA3F2_2"
  OMAPve_y_General_state_of_LKA_function3F2Num/1 -> Index Vector1/3  "OMAPve_y_General_state_of_LKA_function3F2_2"
  Index Vector2/1 -> Bus Creator/2  "OMAPve_g_Coefficient_toregulate_EPS_2"
  Bus Selector1/3 -> Index Vector3/2  "<ELKSve_g_ELK_SWA_Control_convert>"
  OMAPve_g_Column_angle_setpoint3F2Num/1 -> Index Vector3/3  "OMAPve_g_Column_angle_setpoint3F2_2"
  Index Vector3/1 -> Bus Creator/3  "OMAPve_g_Column_angle_setpoint3F2_2"
  Index Vector1/1 -> Bus Creator/1  "OMAPve_y_General_state_of_LKA_function3F2_2"
  Bus Creator/1 -> Out1/1
  In3/1 -> Bus Selector1/1
  Bus Selector2/1 -> Compare To Constant/1  "<AEBSve_d_AEBAlertReq_convert>"
  Compare To Constant4/1 -> Logical Operator1/2
  Compare To Constant/1 -> Logical Operator1/1
  In1/1 -> Bus Selector2/1
  In2/1 -> Bus Selector4/1
  Bus Selector4/1 -> Compare To Constant4/1  "<JABSve_d_DbAlertReq_convert>"

== system OMAP/Runnable_OMAP_10ms_sys/OMAP_Module/Subsystem/EPS_Default_Arbitration/FAPA_arb_ADAS ==
  note: 仲裁内暂时将扭矩接口输出0，即ESA未参与仲裁逻辑，只支持ESA的单功能
  note: 仲裁#21——FAPA与ADAS
      | 1. 关于EMS、ESC、EPS执行器控制：FAPA在控制车辆的工作阶段，无条件优先于ADAS各个功能；在其他情况，则直连ADAS内部原本的仲裁结果
      | 2. 关于仪表显示：维持原本的仲裁策略
      | 3. 选用的表征信号，经IMAP转译后为IMAPve_d_APA_AutoPark_WorkSt
  Input_ICALKA : Inport
  Input_FAPA : Inport  Port=2
  Bus Creator : BusCreator  Inputs=8
  Bus Creator10 : BusCreator  Inputs=5
  Bus Creator11 : BusCreator  Inputs=5
  Bus Selector : BusSelector  OutputSignals=IMAPve_d_APA_AutoPark_WorkSt
  Bus Selector1 : BusSelector  OutputSignals=OMAPve_y_Power_steering_power_cut3F2_2,OMAPve_y_General_state_of_LKA_function3F2_2,OMAPve_g_Coefficient_toregulate_EPS_2,OMAPve_g_Column_angle_setpoint3F2_2,OMAPve_y_Permit_to_know_if_LKA_or_LPA3F2_2
  Bus Selector5 : BusSelector  OutputSignals=OMAPve_y_General_state_of_LKA_function3F2_2,OMAPve_g_Coefficient_toregulate_EPS_2,OMAPve_g_Column_angle_setpoint3F2_2,OMAPve_y_Permit_to_know_if_LKA_or_LPA3F2_2
  Constant : Constant  Value=0  OutDataTypeStr=uint8
  Constant1 : Constant  Value=0  OutDataTypeStr=uint8
  Constant2 : Constant  Value=0  OutDataTypeStr=single
  Constant3 : Constant  Value=0  OutDataTypeStr=uint8
  OMAPve_g_Coefficient_toregulate_EPSNum : Constant  Value=0  OutDataTypeStr=single
  OMAPve_g_Column_angle_setpoint3F2Num : Constant  Value=0  OutDataTypeStr=single
  OMAPve_y_General_state_of_LKA_function3F2Num : Constant  Value=0  OutDataTypeStr=uint8
  OMAPve_y_Permit_to_know_if_LKA_or_LPA3F2Num : Constant  Value=0  OutDataTypeStr=uint8
  OMAPve_y_Power_steering_power_cut3F2Num : Constant  Value=0  OutDataTypeStr=uint8
  Switch : Switch  Criteria=u2 > Threshold
  Arbitration_EPS : Outport
  wires:
  Bus Creator11/1 -> Switch/3  "Arbitration_EPS"
  OMAPve_g_Coefficient_toregulate_EPSNum/1 -> Bus Creator10/3  "OMAPve_g_Coefficient_toregulate_EPS_2"
  Bus Selector5/3 -> Bus Creator11/4  "<OMAPve_g_Column_angle_setpoint3F2_2>"
  OMAPve_y_General_state_of_LKA_function3F2Num/1 -> Bus Creator10/2  "OMAPve_y_General_state_of_LKA_function3F2_2"
  Bus Creator10/1 -> Switch/1  "AEB_EPS"
  Bus Selector/1 -> Switch/2  "<IMAPve_d_APA_AutoPark_WorkSt>"
  OMAPve_y_Power_steering_power_cut3F2Num/1 -> Bus Creator10/1  "OMAPve_y_Power_steering_power_cut3F2_2"
  OMAPve_g_Column_angle_setpoint3F2Num/1 -> Bus Creator10/4  "OMAPve_g_Column_angle_setpoint3F2_2"
  OMAPve_y_Permit_to_know_if_LKA_or_LPA3F2Num/1 -> Bus Creator10/5  "OMAPve_y_Permit_to_know_if_LKA_or_LPA3F2_2"
  Input_FAPA/1 -> Bus Selector/1
  Bus Selector5/2 -> Bus Creator11/3  "<OMAPve_g_Coefficient_toregulate_EPS_2>"
  Constant/1 -> Bus Creator11/1  "OMAPve_y_Power_steering_power_cut3F2_2"
  Bus Selector5/4 -> Bus Creator11/5  "<OMAPve_y_Permit_to_know_if_LKA_or_LPA3F2_2>"
  Bus Selector5/1 -> Bus Creator11/2  "<OMAPve_y_General_state_of_LKA_function3F2_2>"
  Switch/1 -> Bus Selector1/1  "Arbitration_EPS"
  Input_ICALKA/1 -> Bus Selector5/1
  Bus Selector1/1 -> Bus Creator/1  "<OMAPve_y_Power_steering_power_cut3F2_2>"
  Bus Selector1/2 -> Bus Creator/2  "<OMAPve_y_General_state_of_LKA_function3F2_2>"
  Bus Selector1/3 -> Bus Creator/3  "<OMAPve_g_Coefficient_toregulate_EPS_2>"
  Bus Selector1/4 -> Bus Creator/4  "<OMAPve_g_Column_angle_setpoint3F2_2>"
  Bus Selector1/5 -> Bus Creator/5  "<OMAPve_y_Permit_to_know_if_LKA_or_LPA3F2_2>"
  Bus Creator/1 -> Arbitration_EPS/1  "Arbitration_EPS"
  Constant2/1 -> Bus Creator/7  "OMAPve_g_ADAS_ESATorqueReq_2"
  Constant1/1 -> Bus Creator/6  "OMAPve_y_ADAS_ESAState_2"
  Constant3/1 -> Bus Creator/8  "OMAPve_y_ADAS_ESARequest_2"

== system OMAP/Runnable_OMAP_10ms_sys/OMAP_Module/Subsystem/EPS_Default_Arbitration/ICA_arb_LKA ==
  note: 仲裁#6——ICA与LKA/ELK
      | ICA与LKA和ELK的仲裁，关于线控执行器：ICA_STATE不为3且LKA/ELK对EPS的STATE为3或4则LKA/ELK优先，否则ICA优先
  Input_ICA : Inport
  Input_LKAELK : Inport  Port=2
  Bus Creator : BusCreator  Inputs=4
  Bus Selector : BusSelector  OutputSignals=OMAPve_g_Coefficient_toregulate_EPS_2,OMAPve_g_Column_angle_setpoint3F2_2,OMAPve_y_Permit_to_know_if_LKA_or_LPA3F2_2,OMAPve_y_General_state_of_LKA_function3F2_2
  Bus Selector3 : BusSelector  OutputSignals=actuator.ICABve_d_ICAState_convert,actuator.OMAPve_g_Coefficient_toregulate_EPS_2,actuator.ICABve_g_SteerAngleCmd_convert,actuator.OMAPve_y_Permit_to_know_if_LKA_or_LPA3F2_2,actuator.OMAPve_y_General_state_of_LKA_function3F2_2
  Compare To Constant : simulink/Logic and Bit Operations/Compare To Constant  relop=~=  const=3  OutDataTypeStr=boolean
  Compare To Constant1 : simulink/Logic and Bit Operations/Compare To Constant  relop===  const=4  OutDataTypeStr=boolean
  Compare To Constant2 : simulink/Logic and Bit Operations/Compare To Constant  relop===  const=3  OutDataTypeStr=boolean
  Logical Operator : Logic  AllPortsSameDT=off  OutDataTypeStr=boolean
  Logical Operator1 : Logic  Operator=OR  AllPortsSameDT=off  OutDataTypeStr=boolean
  Switch1 : Switch  Criteria=u2 ~= 0  OutDataTypeStr=uint8
  Switch2 : Switch  Criteria=u2 ~= 0  OutDataTypeStr=uint8
  Switch4 : Switch  Criteria=u2 ~= 0  OutDataTypeStr=single
  Switch5 : Switch  Criteria=u2 ~= 0  OutDataTypeStr=single
  Out1 : Outport
  wires:
  Bus Selector3/4 -> Switch2/3  "<OMAPve_y_Permit_to_know_if_LKA_or_LPA3F2_2>"
  Logical Operator/1 -> Switch1/2, Switch2/2, Switch5/2, Switch4/2
  Bus Selector3/5 -> Switch1/3  "<OMAPve_y_General_state_of_LKA_function3F2_2>"
  Switch4/1 -> Bus Creator/1  "OMAPve_g_Coefficient_toregulate_EPS_2"
  Bus Selector3/2 -> Switch4/3  "<OMAPve_g_Coefficient_toregulate_EPS_2>"
  Switch5/1 -> Bus Creator/2  "OMAPve_g_Column_angle_setpoint3F2_2"
  Bus Selector3/3 -> Switch5/3  "<ICABve_g_SteerAngleCmd_convert>"
  Switch1/1 -> Bus Creator/4  "OMAPve_y_General_state_of_LKA_function3F2_2"
  Switch2/1 -> Bus Creator/3  "OMAPve_y_Permit_to_know_if_LKA_or_LPA3F2_2"
  Bus Creator/1 -> Out1/1
  Input_LKAELK/1 -> Bus Selector/1
  Input_ICA/1 -> Bus Selector3/1
  Bus Selector/4 -> Switch1/1, Compare To Constant2/1, Compare To Constant1/1  "<OMAPve_y_General_state_of_LKA_function3F2_2>"
  Bus Selector/1 -> Switch4/1  "<OMAPve_g_Coefficient_toregulate_EPS_2>"
  Bus Selector/2 -> Switch5/1  "<OMAPve_g_Column_angle_setpoint3F2_2>"
  Bus Selector/3 -> Switch2/1  "<OMAPve_y_Permit_to_know_if_LKA_or_LPA3F2_2>"
  Bus Selector3/1 -> Compare To Constant/1  "<ICABve_d_ICAState_convert>"
  Compare To Constant1/1 -> Logical Operator1/1
  Compare To Constant/1 -> Logical Operator/2
  Compare To Constant2/1 -> Logical Operator1/2
  Logical Operator1/1 -> Logical Operator/1

== system OMAP/Runnable_OMAP_10ms_sys/OMAP_Module/Subsystem/EPS_Default_Arbitration/LKA_arb_ELK ==
  note: 仲裁#7——ELK与LKA
      | ELK开关打开且LKA开关关闭时直接输出ELK，其他情况：1、对EPS和车道线显示：默认输出LKA，谁先发出控制指令上升沿便输出谁，直到该功能控制指令消失的标定时间后再重新根据谁先发出控制指令的上升沿来判断输出谁，在标定时间内被输出功能若再次出现控制指令上升沿，则再次响应输出该功能；2、对脱手报警：对LKA与ELK的脱手报警取或
  note: 只有ELK开关打开且LKA开关关闭时，才输出ELK，其他情况下按仲裁#7判断输出
  Input_FDMM : Inport
  Input_LKAS : Inport  Port=2
  Input_ELKS : Inport  Port=3
  AND : Logic  AllPortsSameDT=off  OutDataTypeStr=boolean
  Bus Creator : BusCreator  Inputs=4
  Bus Selector : BusSelector  OutputSignals=LKASve_y_EPS_State_Control_convert,LKASve_g_EPS_Factor_Control_convert,LKASve_g_LKA_SWA_Control_convert,LKASve_y_EPS_LKA_Control_convert
  Bus Selector1 : BusSelector  OutputSignals=OMAPve_y_General_state_of_LKA_function3F2_2,OMAPve_g_Coefficient_toregulate_EPS_2,OMAPve_g_Column_angle_setpoint3F2_2,OMAPve_y_Permit_to_know_if_LKA_or_LPA3F2_2
  Bus Selector2 : BusSelector  OutputSignals=FDMMve_d_ElkFcnConf_convert,FDMMve_d_LkaFcnConf_convert
  Compare To Constant : simulink/Logic and Bit Operations/Compare To Constant  relop===  const=uint16(0)  OutDataTypeStr=boolean
  Compare To Constant1 : simulink/Logic and Bit Operations/Compare To Constant  relop===  const=uint16(1)  OutDataTypeStr=boolean
  Index Vector : MultiPortSwitch  Inputs=2  OutDataTypeStr=uint8
  Index Vector1 : MultiPortSwitch  Inputs=2  OutDataTypeStr=single
  Index Vector2 : MultiPortSwitch  Inputs=2  OutDataTypeStr=single
  Index Vector3 : MultiPortSwitch  Inputs=2  OutDataTypeStr=uint8
  Index Vector4 : MultiPortSwitch  DataPortOrder=Zero-based contiguous  Inputs=2  zeroidx=on  OutDataTypeStr=uint8
  Index Vector5 : MultiPortSwitch  DataPortOrder=Zero-based contiguous  Inputs=2  zeroidx=on  OutDataTypeStr=single
  Index Vector6 : MultiPortSwitch  DataPortOrder=Zero-based contiguous  Inputs=2  zeroidx=on  OutDataTypeStr=single
  Index Vector7 : MultiPortSwitch  DataPortOrder=Zero-based contiguous  Inputs=2  zeroidx=on  OutDataTypeStr=uint8
  Subsystem : Subsystem  Commented=on
  Subsystem2 : Subsystem
  Out1 : Outport
  wires:
  Bus Selector1/4 -> Index Vector7/3, Index Vector3/3  "<OMAPve_y_Permit_to_know_if_LKA_or_LPA3F2_2>"
  Index Vector4/1 -> Bus Creator/1  "OMAPve_y_General_state_of_LKA_function3F2_2"
  Bus Selector1/2 -> Index Vector5/3, Index Vector1/3  "<OMAPve_g_Coefficient_toregulate_EPS_2>"
  Index Vector6/1 -> Bus Creator/3  "OMAPve_g_Column_angle_setpoint3F2_2"
  Bus Selector/4 -> Index Vector3/2  "<LKASve_y_EPS_LKA_Control_convert>"
  Bus Selector1/1 -> Subsystem2/2(<OMAPve_y_General_state_of_LKA_function3F2_2>), Index Vector4/3, Index Vector/3  "<OMAPve_y_General_state_of_LKA_function3F2_2>"
  Bus Selector/2 -> Index Vector1/2  "<LKASve_g_EPS_Factor_Control_convert>"
  Index Vector7/1 -> Bus Creator/4  "OMAPve_y_Permit_to_know_if_LKA_or_LPA3F2_2"
  Index Vector5/1 -> Bus Creator/2  "OMAPve_g_Coefficient_toregulate_EPS_2"
  Bus Selector/1 -> Subsystem2/1(<LKASve_y_EPS_State_Control_convert>), Index Vector/2  "<LKASve_y_EPS_State_Control_convert>"
  Bus Selector1/3 -> Index Vector6/3, Index Vector2/3  "<OMAPve_g_Column_angle_setpoint3F2_2>"
  Bus Selector/3 -> Index Vector2/2  "<LKASve_g_LKA_SWA_Control_convert>"
  Input_LKAS/1 -> Bus Selector/1
  Bus Creator/1 -> Out1/1
  Input_ELKS/1 -> Bus Selector1/1
  Index Vector/1 -> Index Vector4/2  "OMAPve_y_General_state_of_LKA_function3F2_2"
  Index Vector1/1 -> Index Vector5/2  "OMAPve_g_Coefficient_toregulate_EPS_2"
  Index Vector2/1 -> Index Vector6/2  "OMAPve_g_Column_angle_setpoint3F2_2"
  Index Vector3/1 -> Index Vector7/2  "OMAPve_y_Permit_to_know_if_LKA_or_LPA3F2_2"
  Subsystem2/1(state) -> Index Vector3/1, Index Vector2/1, Index Vector1/1, Index Vector/1
  Bus Selector2/1 -> Compare To Constant1/1  "<FDMMve_d_ElkFcnConf_convert>"
  Bus Selector2/2 -> Compare To Constant/1  "<FDMMve_d_LkaFcnConf_convert>"
  Input_FDMM/1 -> Bus Selector2/1
  Compare To Constant/1 -> AND/2
  Compare To Constant1/1 -> AND/1
  AND/1 -> Index Vector7/1, Index Vector6/1, Index Vector5/1, Index Vector4/1
